simulink model "output_windows"  (R2021a)
settings: Solver=VariableStepAuto  StartTime=0.0  StopTime=3  RelTol=1e-3
settings Model: SimulationMode=accelerator  Creator=chigo  LastModifiedBy=chigo

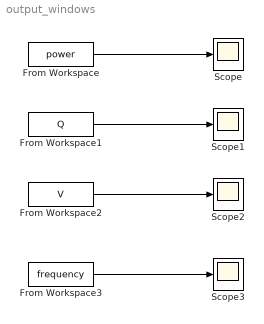
== system output_windows ==
  From Workspace : FromWorkspace  VariableName=power  SampleTime=0.0005
  From Workspace1 : FromWorkspace  VariableName=Q  SampleTime=0.0005
  From Workspace2 : FromWorkspace  VariableName=V  SampleTime=0.0005
  From Workspace3 : FromWorkspace  VariableName=frequency  SampleTime=0.0005
  Scope{,1..3} (4 alike) : Scope
  wires:
  From Workspace/1 -> Scope/1
  From Workspace1/1 -> Scope1/1
  From Workspace2/1 -> Scope2/1
  From Workspace3/1 -> Scope3/1
